simulink model "SingleTank"  (Simulink 9.3)
settings: Solver=ode5  StartTime=0.0  StopTime=1000  FixedStep=1  MaxStep=0.1  RelTol=1e-3
StopFcn:
  | %plot_sim_data
Description:
  | The model describes dynamic properties of tank level system. The differential equation is:
  |                                            d/dt{Ah(t))=ku(t)-a*sqrt(2*g*h(t))
settings Model: Creator=Huynh Thai Hoang  LastModifiedBy=forev  ExtModeTrigMode=oneshot  ExtModeArmWhenConnect=off
settings SolverCC: InitialStep=0.1
settings DataIOCC: SaveOutput=off  SaveTime=off  SignalLoggingName=sigsOut
settings OptimizationCC: BooleanDataType=off  ExpressionDepthLimit=2147483647
settings DebuggingCC: SaveWithParameterizedLinksMsg=none  SignalResolutionControl=TryResolveAllWithWarning  MultiTaskDSMMsg=warning  MultiTaskCondExecSysMsg=none  StateNameClashWarn=warning
settings HardwareCC: TargetUnknown=on
settings GRTTargetCC: GeneratePreprocessorConditionals=Disable all

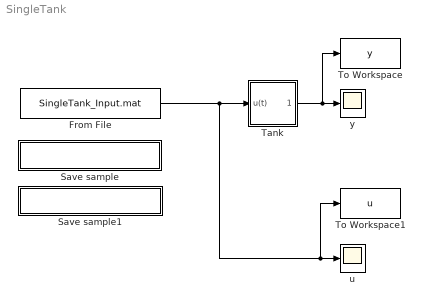
== system SingleTank ==
  From File : FromFile  FileName=SingleTank_Input.mat  SampleTime=0
  Save sample : Subsystem
      settings: OpenFcn=save_sample
      mask Display: disp('Save sampled data')
  Save sample1 : Subsystem
      settings: OpenFcn=signal_gen
      mask Display: disp('Generate Random Input')
  Tank : Subsystem  mask{A1=200, A2=150, b1=1, b2=1, g=9.81, h1_max=inf, C=0.8, h2_max=100}
      mask init:
      | g=981;
      mask Display:
      | plot([0.1 0.3 0.9],[0.9 0.1 0.1]);
      | plot([0.9 0.7 0.9],[0.9 0.2 0.2]);
  To Workspace : ToWorkspace  VariableName=y  SampleTime=-1
  To Workspace1 : ToWorkspace  VariableName=u  SampleTime=-1
  u : Scope
  y : Scope
  wires:
  Tank/1(y2(t)) -> To Workspace/1, y/1
  From File/1 -> Tank/1(u(t)), To Workspace1/1, u/1

== system SingleTank/Save sample ==

== system SingleTank/Save sample1 ==

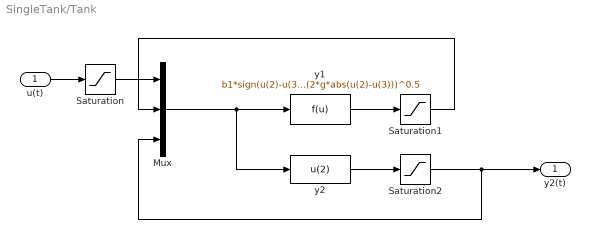
== system SingleTank/Tank ==
  u(t) : Inport
  Mux : Mux  Inputs=3
  Saturation : Saturate  UpperLimit=50  LowerLimit=0
  Saturation1 : Saturate  UpperLimit=h1_max  LowerLimit=0
  Saturation2 : Saturate  UpperLimit=h2_max  LowerLimit=0
  y1 : Fcn  Expr=b1*sign(u(2)-u(3))*(2*g*abs(u(2)-u(3)))^0.5
  y2 : Fcn  Expr=u(2)
  y2(t) : Outport
  wires:
  u(t)/1 -> Saturation/1
  Mux/1 -> y2/1, y1/1
  Saturation/1 -> Mux/1
  y1/1 -> Saturation1/1
  Saturation1/1 -> Mux/2
  y2/1 -> Saturation2/1
  Saturation2/1 -> Mux/3, y2(t)/1
